simulink library "AveragingFilter"  (R2019b)
settings: Solver=VariableStepAuto  StartTime=0.0  StopTime=10.0  RelTol=1e-3
settings Model: Creator=Nick  LastModifiedBy=Nick
settings DataIOCC: ReturnWorkspaceOutputs=off
settings DebuggingCC: ArithmeticOperatorsInVariantConditions=warning
settings SFSimCC: CustomCodeUndefinedFunction=UseInterfaceOnly

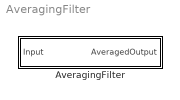
== system AveragingFilter ==
  AveragingFilter : Subsystem  TreatAsAtomicUnit=on  mask{factor=10}
      mask Display:
      | color('blue');
      | disp(sprintf(['Averaging Filter\n', num2str(factor), 'x']));

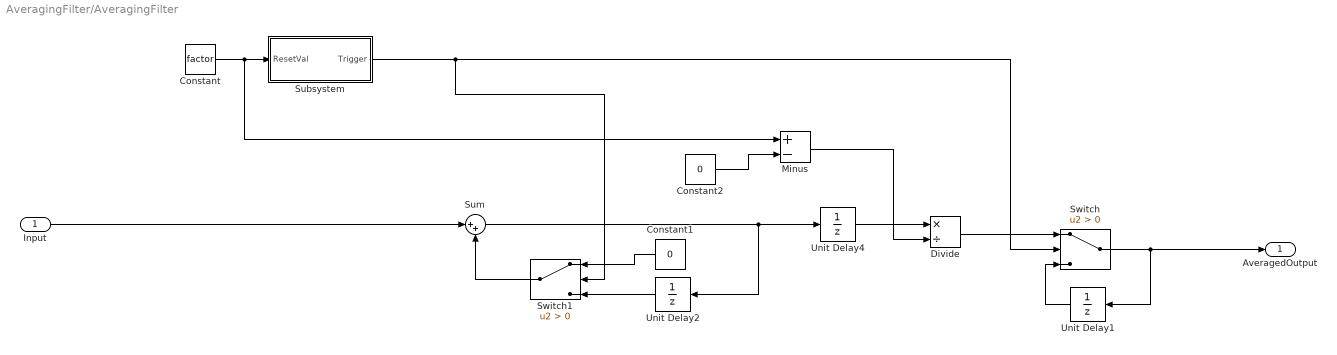
== system AveragingFilter/AveragingFilter ==
  Input : Inport
  Constant : Constant  Value=factor
  Constant1 : Constant  Value=0
  Constant2 : Constant  Value=0
  Divide : Product  Inputs=*/
  Minus : Sum  Inputs=+-
  Subsystem : Subsystem
  Sum : Sum  Inputs=|++
  Switch : Switch  Criteria=u2 > Threshold
  Switch1 : Switch  Criteria=u2 > Threshold
  Unit Delay1 : UnitDelay  SampleTime=-1  HasFrameUpgradeWarning=on
  Unit Delay2 : UnitDelay  SampleTime=-1  HasFrameUpgradeWarning=on
  Unit Delay4 : UnitDelay  SampleTime=-1  HasFrameUpgradeWarning=on
  AveragedOutput : Outport
  wires:
  Switch/1 -> Unit Delay1/1, AveragedOutput/1
  Unit Delay1/1 -> Switch/3
  Constant/1 -> Minus/1, Subsystem/1(ResetVal)
  Input/1 -> Sum/1
  Switch1/1 -> Sum/2
  Unit Delay2/1 -> Switch1/3
  Constant1/1 -> Switch1/1
  Divide/1 -> Switch/1
  Sum/1 -> Unit Delay4/1, Unit Delay2/1
  Subsystem/1(Trigger) -> Switch1/2, Switch/2
  Unit Delay4/1 -> Divide/1
  Minus/1 -> Divide/2
  Constant2/1 -> Minus/2

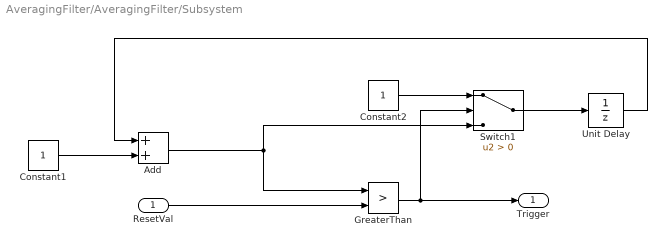
== system AveragingFilter/AveragingFilter/Subsystem ==
  ResetVal : Inport
  Add : Sum
  Constant1 : Constant
  Constant2 : Constant
  GreaterThan : RelationalOperator  Operator=>  OutDataTypeStr=boolean  RndMeth=Simplest
  Switch1 : Switch  Criteria=u2 > Threshold
  Unit Delay : UnitDelay  SampleTime=-1  HasFrameUpgradeWarning=on
  Trigger : Outport
  wires:
  Add/1 -> GreaterThan/1, Switch1/3
  Unit Delay/1 -> Add/1
  GreaterThan/1 -> Trigger/1, Switch1/2
  Switch1/1 -> Unit Delay/1
  ResetVal/1 -> GreaterThan/2
  Constant2/1 -> Switch1/1
  Constant1/1 -> Add/2
